simulink model "EXP7_Part1"  (R2018a)
settings: Solver=VariableStepAuto  StartTime=0.0  StopTime=4  RelTol=1e-3
libraries: dsparch4 x1
settings Model: Creator=user  LastModifiedBy=shohan

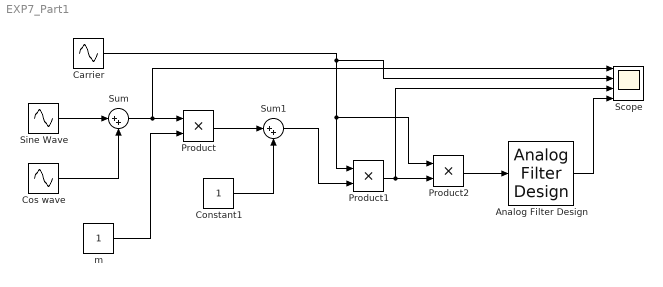
== system EXP7_Part1 ==
  Analog Filter Design : dsparch4/Analog Filter Design  method=Butterworth  filttype=Lowpass  N=8  Wlo=2*pi*10  Whi=80  Rp=2  Rs=40
  Carrier : Sin  Frequency=2*pi*50  Phase=pi/2  SampleTime=1/5000
  Constant1 : Constant
  Cos wave : Sin  Amplitude=3  Frequency=2*pi*6  Phase=pi/2  SampleTime=1/5000
  Product : Product
  Product1 : Product
  Product2 : Product
  Scope : Scope  NumInputPorts=4
  Sine Wave : Sin  Amplitude=2  Frequency=2*pi*4  SampleTime=1/5000
  Sum : Sum  Inputs=|++
  Sum1 : Sum  Inputs=|++
  m : Constant
  wires:
  Cos wave/1 -> Sum/2
  Sine Wave/1 -> Sum/1
  Sum/1 -> Scope/1, Product/1
  m/1 -> Product/2
  Product/1 -> Sum1/1
  Constant1/1 -> Sum1/2
  Sum1/1 -> Product1/2
  Carrier/1 -> Scope/2, Product2/1, Product1/1
  Product1/1 -> Scope/3, Product2/2
  Product2/1 -> Analog Filter Design/1
  Analog Filter Design/1 -> Scope/4
